simulink model "KalmanFilter"  (R2024a)
settings: Solver=VariableStepAuto  StartTime=0.0  StopTime=10.0  RelTol=1e-3
undefined symbols (not defined in the file or in its folder): Ad, Bd, C, D, GQG, P0, R, x0
libraries: sdl_lib x10, nesl_utility x6, fl_lib x4
settings Model: Creator=Z634594  LastModifiedBy=marisao
settings SolverCC: AlgebraicLoopSolver=TrustRegion
settings DebuggingCC: UnconnectedInputMsg=warning  UnconnectedOutputMsg=warning  UnconnectedLineMsg=warning
settings ModelReferenceCC: EnableRefExpFcnMdlSchedulingChecks=on
settings SFSimCC: CustomCodeUndefinedFunction=UseInterfaceOnly
settings RTWCC: GPUComputeCapability=3.5

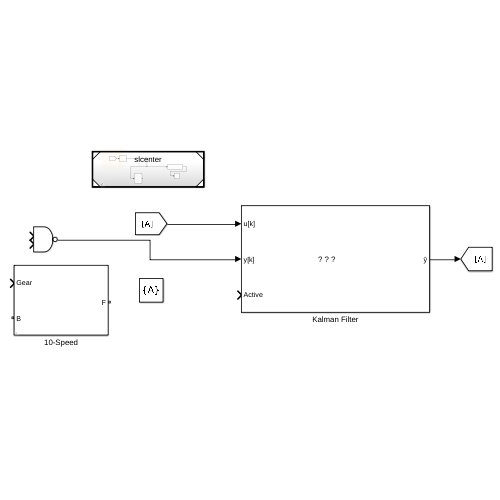
[thumbnail: Simulink's stored preview of the top-level diagram]
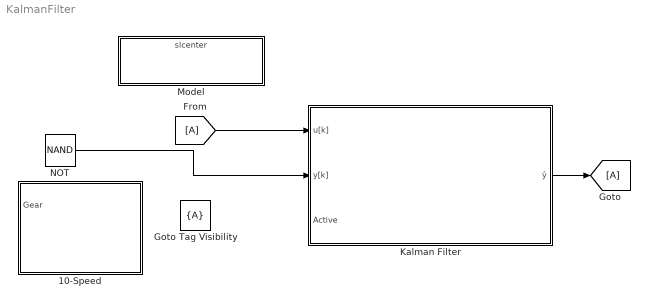
== system KalmanFilter ==
  10-Speed : Subsystem  mask(10-Speed){InitGear=Neutral, ShowInLibBrowser=0, ClutchSchedule={[0 1 1 1 0 1];[0 1 1 0 1 1];[0 1 0 1 1 1];[0 0 1 1 1 1];[1 0 0 1 1 1];[1 0 1 0 1 1];[1 0 1 1 0 1];[1 0 1 1 1 0];[1 1 1 1 0 0];[1 1 0 1 1 0];[1 1 0 1 0 1];[1 1 0 1 0 0]}}
      mask prompts: InitGear "Initial gear"
      mask help: physmod:sdl:library:transmissions:TenSpeed
      mask init:
      | set_param([gcb,'/Clutch A'],'initial_state_locked',num2str(ClutchSchedule{InitGear}(1)));
      | set_param([gcb,'/Clutch B'],'initial_state_locked',num2str(ClutchSchedule{InitGear}(2)));
      | set_param([gcb,'/Clutch C'],'initial_state_locked',num2str(ClutchSchedule{InitGear}(3)));
      | set_param([gcb,'/Clutch D'],'initial_state_locked',num2str(ClutchSchedule{InitGear}(4)));
      | set_param([gcb,'/Clutch E'],'initial_state_locked',num2str(ClutchSchedule{InitGear}(5)));
      | set_param([gcb,'/Clutch F'],'initial_state_locked',num2str(ClutchSchedule{InitGear}(6)));
      mask Help: web([docroot '/sdl/ref/10speed.html'])
      mask TypeOptions InitGear: 10 | 9 | 8 | 7 | 6 | 5 | 4 | 3 | 2 | 1 | physmod:sdl:library:transmissions:Reverse | physmod:sdl:library:transmissions:Neutral
  From : From
  Goto : Goto
  Goto Tag Visibility : GotoTagVisibility
  Kalman Filter : Subsystem
      mask Display: image('C:\Users\Z634594\OneDrive - ZF Friedrichshafen AG\Workspace_MATLAB\14_Tj-Measurement\KalmanFilter\KalmanFilter\img\Kalman.png');
  Model : ModelReference  ModelNameDialog=slcenter.slx  SimulationMode=Normal  ModelReferenceVersion=1.1
  NOT : Logic  Operator=NAND  IconShape=distinctive  AllPortsSameDT=off  OutDataTypeStr=boolean
  wires:
  Kalman Filter/1(ŷ) -> Goto/1
  From/1 -> Kalman Filter/1(u[k])
  NOT/1 -> Kalman Filter/2(y[k])

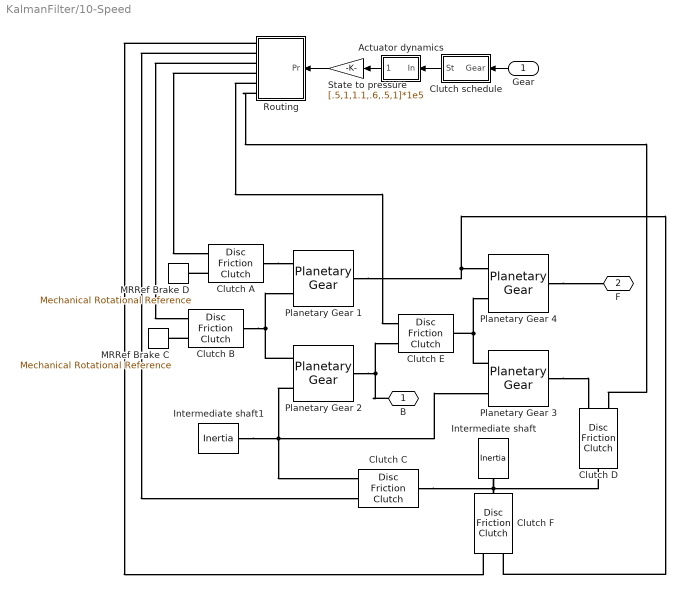
== system KalmanFilter/10-Speed ==
  Gear : Inport
  Actuator dynamics : Subsystem  mask(First-order lag supporting vector signals){b=[1 1 1 1 1 1]*0.05, x_initial=ClutchSchedule{InitGear}}
      mask prompts: b "Filter time constant"; x_initial "Initial output"
      mask help: Models a lag of the form 1/(b*s+1) where s is the Laplace operator.
  Clutch schedule : Subsystem
  Clutch A : sdl_lib/Clutches/Disc Friction Clutch  geometry_model=1  r_eff=130 mm  d_o=150 mm  d_i=100 mm  nS=3  piston_area=0.001 m^2  unidirectional=0  enable_faults=simscape.enum.onoff.off  fault_type=sdl.enum.clutchFault.lock  friction_model=1  mu_w_vector=[0, 100, 1000] rad/s  temperature_TLU=[280, 300, 320] K  mu_static=0.35  mu_static_vector=[.4, .38, .36]  mu_coulomb=0.3  mu_coulomb_vector=[.3, .22, .19]  mu_coulomb_temp_vector=[.3, .28, .25]  mu_coulomb_matrix=[.34, .32, .3; .3, .28, .25; .25, .2, .15]  mu_interp_method=simscape.enum.interpolation.linear  mu_extrap_method=simscape.enum.extrapolation.linear  d_f=1  w_tol=0.001 rad/s  pressure_min=100 Pa  mu_visc=0 N*m/(rad/s)  initial_state_locked=1  thermal_mass=25 kJ/K  T_init=300 K
      settings: InternalSimscapePortConfiguration="{\"Bottom\":[],\"Left\":[{\"id\":\"P\",\"label\":\"P\",\"type\":\"input\"},{\"id\":\"B\",\"label\":\"B\",\"type\":\"foundation.mechanical.rotational.rotational\"}],\"Right\":[{\"id\":\"F\",\"label\":\"F\",\"type\":\"foundation.mechanical.rotational.rotational\"}],\"Top\":[]}"
  Clutch B : sdl_lib/Clutches/Disc Friction Clutch  geometry_model=1  r_eff=130 mm  d_o=150 mm  d_i=100 mm  nS=5  piston_area=0.001 m^2  unidirectional=0  enable_faults=simscape.enum.onoff.off  fault_type=sdl.enum.clutchFault.lock  friction_model=1  mu_w_vector=[0, 100, 1000] rad/s  temperature_TLU=[280, 300, 320] K  mu_static=0.35  mu_static_vector=[.4, .38, .36]  mu_coulomb=0.3  mu_coulomb_vector=[.3, .22, .19]  mu_coulomb_temp_vector=[.3, .28, .25]  mu_coulomb_matrix=[.34, .32, .3; .3, .28, .25; .25, .2, .15]  mu_interp_method=simscape.enum.interpolation.linear  mu_extrap_method=simscape.enum.extrapolation.linear  d_f=1  w_tol=0.001 rad/s  pressure_min=100 Pa  mu_visc=0 N*m/(rad/s)  initial_state_locked=1  thermal_mass=25 kJ/K  T_init=300 K
      settings: InternalSimscapePortConfiguration="{\"Bottom\":[],\"Left\":[{\"id\":\"P\",\"label\":\"P\",\"type\":\"input\"},{\"id\":\"B\",\"label\":\"B\",\"type\":\"foundation.mechanical.rotational.rotational\"}],\"Right\":[{\"id\":\"F\",\"label\":\"F\",\"type\":\"foundation.mechanical.rotational.rotational\"}],\"Top\":[]}"
  Clutch C : sdl_lib/Clutches/Disc Friction Clutch  geometry_model=1  r_eff=130 mm  d_o=150 mm  d_i=100 mm  nS=5  piston_area=0.001 m^2  unidirectional=0  enable_faults=simscape.enum.onoff.off  fault_type=sdl.enum.clutchFault.lock  friction_model=1  mu_w_vector=[0, 100, 1000] rad/s  temperature_TLU=[280, 300, 320] K  mu_static=0.35  mu_static_vector=[.4, .38, .36]  mu_coulomb=0.3  mu_coulomb_vector=[.3, .22, .19]  mu_coulomb_temp_vector=[.3, .28, .25]  mu_coulomb_matrix=[.34, .32, .3; .3, .28, .25; .25, .2, .15]  mu_interp_method=simscape.enum.interpolation.linear  mu_extrap_method=simscape.enum.extrapolation.linear  d_f=1  w_tol=0.001 rad/s  pressure_min=100 Pa  mu_visc=0 N*m/(rad/s)  initial_state_locked=0  thermal_mass=25 kJ/K  T_init=300 K
      settings: InternalSimscapePortConfiguration="{\"Bottom\":[],\"Left\":[{\"id\":\"P\",\"label\":\"P\",\"type\":\"input\"},{\"id\":\"B\",\"label\":\"B\",\"type\":\"foundation.mechanical.rotational.rotational\"}],\"Right\":[{\"id\":\"F\",\"label\":\"F\",\"type\":\"foundation.mechanical.rotational.rotational\"}],\"Top\":[]}"
  Clutch D : sdl_lib/Clutches/Disc Friction Clutch  geometry_model=1  r_eff=130 mm  d_o=150 mm  d_i=100 mm  nS=6  piston_area=0.001 m^2  unidirectional=0  enable_faults=simscape.enum.onoff.off  fault_type=sdl.enum.clutchFault.lock  friction_model=1  mu_w_vector=[0, 100, 1000] rad/s  temperature_TLU=[280, 300, 320] K  mu_static=0.35  mu_static_vector=[.4, .38, .36]  mu_coulomb=0.3  mu_coulomb_vector=[.3, .22, .19]  mu_coulomb_temp_vector=[.3, .28, .25]  mu_coulomb_matrix=[.34, .32, .3; .3, .28, .25; .25, .2, .15]  mu_interp_method=simscape.enum.interpolation.linear  mu_extrap_method=simscape.enum.extrapolation.linear  d_f=1  w_tol=0.001 rad/s  pressure_min=100 Pa  mu_visc=0 N*m/(rad/s)  initial_state_locked=1  thermal_mass=25 kJ/K  T_init=300 K
      settings: InternalSimscapePortConfiguration="{\"Bottom\":[],\"Left\":[{\"id\":\"P\",\"label\":\"P\",\"type\":\"input\"},{\"id\":\"B\",\"label\":\"B\",\"type\":\"foundation.mechanical.rotational.rotational\"}],\"Right\":[{\"id\":\"F\",\"label\":\"F\",\"type\":\"foundation.mechanical.rotational.rotational\"}],\"Top\":[]}"
  Clutch E : sdl_lib/Clutches/Disc Friction Clutch  geometry_model=1  r_eff=130 mm  d_o=150 mm  d_i=100 mm  nS=5  piston_area=0.001 m^2  unidirectional=0  enable_faults=simscape.enum.onoff.off  fault_type=sdl.enum.clutchFault.lock  friction_model=1  mu_w_vector=[0, 100, 1000] rad/s  temperature_TLU=[280, 300, 320] K  mu_static=0.35  mu_static_vector=[.4, .38, .36]  mu_coulomb=0.3  mu_coulomb_vector=[.3, .22, .19]  mu_coulomb_temp_vector=[.3, .28, .25]  mu_coulomb_matrix=[.34, .32, .3; .3, .28, .25; .25, .2, .15]  mu_interp_method=simscape.enum.interpolation.linear  mu_extrap_method=simscape.enum.extrapolation.linear  d_f=1  w_tol=0.001 rad/s  pressure_min=100 Pa  mu_visc=0 N*m/(rad/s)  initial_state_locked=0  thermal_mass=25 kJ/K  T_init=300 K
      settings: InternalSimscapePortConfiguration="{\"Bottom\":[],\"Left\":[{\"id\":\"P\",\"label\":\"P\",\"type\":\"input\"},{\"id\":\"B\",\"label\":\"B\",\"type\":\"foundation.mechanical.rotational.rotational\"}],\"Right\":[{\"id\":\"F\",\"label\":\"F\",\"type\":\"foundation.mechanical.rotational.rotational\"}],\"Top\":[]}"
  Clutch F : sdl_lib/Clutches/Disc Friction Clutch  geometry_model=1  r_eff=130 mm  d_o=150 mm  d_i=100 mm  nS=4  piston_area=0.001 m^2  unidirectional=0  enable_faults=simscape.enum.onoff.off  fault_type=sdl.enum.clutchFault.lock  friction_model=1  mu_w_vector=[0, 100, 1000] rad/s  temperature_TLU=[280, 300, 320] K  mu_static=0.35  mu_static_vector=[.4, .38, .36]  mu_coulomb=0.3  mu_coulomb_vector=[.3, .22, .19]  mu_coulomb_temp_vector=[.3, .28, .25]  mu_coulomb_matrix=[.34, .32, .3; .3, .28, .25; .25, .2, .15]  mu_interp_method=simscape.enum.interpolation.linear  mu_extrap_method=simscape.enum.extrapolation.linear  d_f=1  w_tol=0.001 rad/s  pressure_min=100 Pa  mu_visc=0 N*m/(rad/s)  initial_state_locked=0  thermal_mass=25 kJ/K  T_init=300 K
      settings: InternalSimscapePortConfiguration="{\"Bottom\":[],\"Left\":[{\"id\":\"P\",\"label\":\"P\",\"type\":\"input\"},{\"id\":\"B\",\"label\":\"B\",\"type\":\"foundation.mechanical.rotational.rotational\"}],\"Right\":[{\"id\":\"F\",\"label\":\"F\",\"type\":\"foundation.mechanical.rotational.rotational\"}],\"Top\":[]}"
  Intermediate shaft : fl_lib/Mechanical/Rotational Elements/Inertia  inertia=0.01 kg*m^2  num_ports=foundation.enum.numPorts2.one  w_specify=off  w_priority=High  w=0 rad/s  w_nominal_specify=off  w_nominal_value=1  w_nominal_unit=rad/s  t_specify=off  t_priority=High  t=0 N*m  t_nominal_specify=off  t_nominal_value=1  t_nominal_unit=N*m
  Intermediate shaft1 : fl_lib/Mechanical/Rotational Elements/Inertia  inertia=0.01 kg*m^2  num_ports=foundation.enum.numPorts2.one  w_specify=off  w_priority=High  w=0 rad/s  w_nominal_specify=off  w_nominal_value=1  w_nominal_unit=rad/s  t_specify=off  t_priority=High  t=0 N*m  t_nominal_specify=off  t_nominal_value=1  t_nominal_unit=N*m
  MRRef Brake C : fl_lib/Mechanical/Rotational Elements/Mechanical Rotational Reference
  MRRef Brake D : fl_lib/Mechanical/Rotational Elements/Mechanical Rotational Reference
  Planetary Gear 1 : sdl_lib/Gears/Planetary Gear  rs_ratio=92/44  friction_model=1  efficiency=[ 0.96 0.98 ]  temperature_TLU=[ 280 300 320 ] K  efficiency_sp_TLU=[ 0.95 0.9 0.85 ]  efficiency_rp_TLU=[ 0.95 0.9 0.85 ]  pwr_thr=[ 0.001 0.001 ] W  mu_visc=[ 0 0 ] N*m/(rad/s)  model_inertia=0  planet_inertia=0.001 kg*m^2  thermal_mass=50 J/K  T_init=300 K
  Planetary Gear 2 : sdl_lib/Gears/Planetary Gear  rs_ratio=89/51  friction_model=1  efficiency=[ 0.96 0.98 ]  temperature_TLU=[ 280 300 320 ] K  efficiency_sp_TLU=[ 0.95 0.9 0.85 ]  efficiency_rp_TLU=[ 0.95 0.9 0.85 ]  pwr_thr=[ 0.001 0.001 ] W  mu_visc=[ 0 0 ] N*m/(rad/s)  model_inertia=0  planet_inertia=0.001 kg*m^2  thermal_mass=50 J/K  T_init=300 K
  Planetary Gear 3 : sdl_lib/Gears/Planetary Gear  rs_ratio=101/63  friction_model=1  efficiency=[ 0.96 0.98 ]  temperature_TLU=[ 280 300 320 ] K  efficiency_sp_TLU=[ 0.95 0.9 0.85 ]  efficiency_rp_TLU=[ 0.95 0.9 0.85 ]  pwr_thr=[ 0.001 0.001 ] W  mu_visc=[ 0 0 ] N*m/(rad/s)  model_inertia=0  planet_inertia=0.001 kg*m^2  thermal_mass=50 J/K  T_init=300 K
  Planetary Gear 4 : sdl_lib/Gears/Planetary Gear  rs_ratio=85/23  friction_model=1  efficiency=[ 0.96 0.98 ]  temperature_TLU=[ 280 300 320 ] K  efficiency_sp_TLU=[ 0.95 0.9 0.85 ]  efficiency_rp_TLU=[ 0.95 0.9 0.85 ]  pwr_thr=[ 0.001 0.001 ] W  mu_visc=[ 0 0 ] N*m/(rad/s)  model_inertia=0  planet_inertia=0.001 kg*m^2  thermal_mass=50 J/K  T_init=300 K
  Routing : Subsystem
  State to pressure : Gain  Gain=[.5,1,1.1,.6,.5,1]*1e5
  B : PMIOPort  Side=Left
  F : PMIOPort  Port=2  Side=Right
  wires:
  Gear/1 -> Clutch schedule/1(Gear)
  Clutch schedule/1(St) -> Actuator dynamics/1(In)
  State to pressure/1 -> Routing/1(Pr)
  Actuator dynamics/1(Out) -> State to pressure/1
  connections:
  Clutch A/LConn2 -- MRRef Brake D/LConn1
  Clutch B/LConn2 -- MRRef Brake C/LConn1
  Planetary Gear 4/LConn1 -- F/RConn1
  B/RConn1 -- Planetary Gear 2/LConn1 -- Clutch E/LConn2
  Clutch A/RConn1 -- Planetary Gear 1/RConn1
  Clutch B/RConn1 -- Planetary Gear 2/RConn2 -- Planetary Gear 1/RConn2
  Planetary Gear 1/LConn1 -- Planetary Gear 4/RConn1 -- Clutch F/LConn2
  Planetary Gear 2/RConn1 -- Intermediate shaft1/LConn1 -- Planetary Gear 3/RConn2 -- Clutch C/LConn2
  Planetary Gear 3/RConn1 -- Planetary Gear 4/RConn2 -- Clutch E/RConn1
  Planetary Gear 3/LConn1 -- Clutch D/LConn2
  Clutch F/RConn1 -- Clutch C/RConn1 -- Intermediate shaft/LConn1 -- Clutch D/RConn1
  Routing/RConn1 -- Clutch F/LConn1
  Routing/RConn2 -- Clutch C/LConn1
  Routing/RConn3 -- Clutch B/LConn1
  Routing/RConn4 -- Clutch A/LConn1
  Routing/RConn5 -- Clutch E/LConn1
  Routing/RConn6 -- Clutch D/LConn1

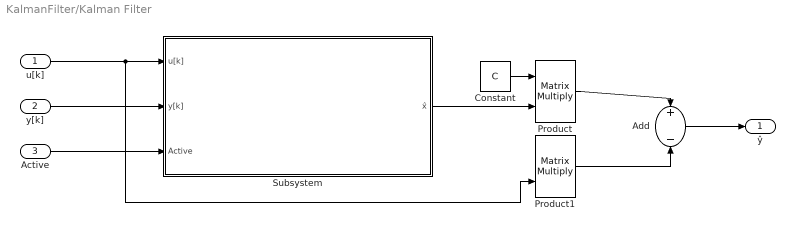
== system KalmanFilter/Kalman Filter ==
  u[k] : Inport
  y[k] : Inport  Port=2
  Active : Inport  Port=3
  Add : Sum  Inputs=+-
  Constant : Constant  Value=C  VectorParams1D=off
  Product : Product  Multiplication=Matrix(*)
  Product1 : Product  Multiplication=Matrix(*)
  Subsystem : Subsystem
      mask Display: image('C:\Users\Z634594\OneDrive - ZF Friedrichshafen AG\Workspace_MATLAB\14_Tj-Measurement\KalmanFilter\KalmanFilter\img\KalmanEquations.jpg');
  ŷ : Outport  VectorParamsAs1DForOutWhenUnconnected=off
  wires:
  u[k]/1 -> Product1/2, Subsystem/1(u[k])
  y[k]/1 -> Subsystem/2(y[k])
  ? -> Product1/1
  Product/1 -> Add/1
  Constant/1 -> Product/1
  Subsystem/1(x̂) -> Product/2
  Add/1 -> ŷ/1
  Product1/1 -> Add/2
  Active/1 -> Subsystem/3(Active)

== system KalmanFilter/10-Speed/Actuator dynamics ==
  In : Inport
  Gain : Gain  Gain=1./b
  Integrator : Integrator  InitialCondition=x_initial.*b
  Sum : Sum  Inputs=|+-  InputSameDT=on  SaturateOnIntegerOverflow=on  OutDataTypeStr=Inherit: Same as first input
  Out : Outport  VectorParamsAs1DForOutWhenUnconnected=off
  wires:
  Gain/1 -> Out/1, Sum/2
  Integrator/1 -> Gain/1
  In/1 -> Sum/1
  Sum/1 -> Integrator/1

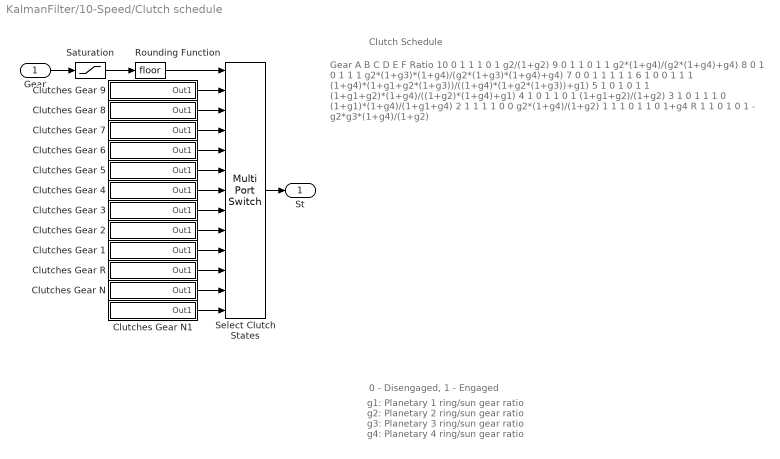
== system KalmanFilter/10-Speed/Clutch schedule ==
  note: Clutch Schedule
  note: Gear
      | A
      | B
      | C
      | D
      | E
      | F
      | Ratio
      |
      | 10
      | 0
      | 1
      | 1
      | 1
      | 0
      | 1
      | g2/(1+g2)
      |
      | 9
      | 0
      | 1
      | 1
      | 0
      | 1
      | 1
      | g2*(1+g4)/(g2*(1+g4)+g4)
      |
      | 8
      | 0
      | 1
      | 0
      | 1
      | 1
      | 1
      | g2*(1+g3)*(1+g4)/(g2*(1+g3)*(1+g4)+g4)
      |
      | 7
      | 0
      | 0
      | 1
      | 1
      | 1
      | 1
      | 1
      |
      | 6
      | 1
      | 0
      | 0
      | 1
      | 1
      | 1
      | (1+g4)*(1+g1+g2*(1+g3))/((1+g4)*(1+g2*(1+g3))+g1)
      |
      | 5
      | 1
      | 0
      | 1
      | 0
      | 1
      | 1
      | (1+g1+g2)*(1+g4)/((1+g2)*(1+g4)+g1)
      |
      | 4
      | 1
      | 0
      | 1
      | 1
      | 0
      | 1
      | (1+g1+g2)/(1+g2)
      |
      | 3
      | 1
      | 0
      | 1
      | 1
      | 1
      | 0
      | (1+g1)*(1+g4)/(1+g1+g4)
      |
      | 2
      | 1
      | 1
      | 1
      | 1
      | 0
      | 0
      | g2*(1+g4)/(1+g2)
      |
      | 1
      | 1
      | 1
      | 0
      | 1
      | 1
      | 0
      | 1+g4
      |
      | R
      | 1
      | 1
      | 0
      | 1
      | 0
      | 1
      | - g2*g3*(1+g4)/(1+g2)
  note: 0 - Disengaged, 1 - Engaged
  note: g1: Planetary 1 ring/sun gear ratio
      | g2: Planetary 2 ring/sun gear ratio
      | g3: Planetary 3 ring/sun gear ratio
      | g4: Planetary 4 ring/sun gear ratio
  Gear : Inport
  Clutches Gear 1 : Subsystem  mask{Clutches=ClutchSchedule{9}}
      settings: OpenFcn=open_system(gcb,'force');
      mask Display: disp(Clutches)
  Clutches Gear 2 : Subsystem  mask{Clutches=ClutchSchedule{8}}
      settings: OpenFcn=open_system(gcb,'force');
      mask Display: disp(Clutches)
  Clutches Gear 3 : Subsystem  mask{Clutches=ClutchSchedule{7}}
      settings: OpenFcn=open_system(gcb,'force');
      mask Display: disp(Clutches)
  Clutches Gear 4 : Subsystem  mask{Clutches=ClutchSchedule{6}}
      settings: OpenFcn=open_system(gcb,'force');
      mask Display: disp(Clutches)
  Clutches Gear 5 : Subsystem  mask{Clutches=ClutchSchedule{5}}
      settings: OpenFcn=open_system(gcb,'force');
      mask Display: disp(Clutches)
  Clutches Gear 6 : Subsystem  mask{Clutches=ClutchSchedule{4}}
      settings: OpenFcn=open_system(gcb,'force');
      mask Display: disp(Clutches)
  Clutches Gear 7 : Subsystem  mask{Clutches=ClutchSchedule{3}}
      settings: OpenFcn=open_system(gcb,'force');
      mask Display: disp(Clutches)
  Clutches Gear 8 : Subsystem  mask{Clutches=ClutchSchedule{2}}
      settings: OpenFcn=open_system(gcb,'force');
      mask Display: disp(Clutches)
  Clutches Gear 9 : Subsystem  mask{Clutches=ClutchSchedule{1}}
      settings: OpenFcn=open_system(gcb,'force');
      mask Display: disp(Clutches)
  Clutches Gear N : Subsystem  mask{Clutches=ClutchSchedule{11}}
      settings: OpenFcn=open_system(gcb,'force');
      mask Display: disp(Clutches)
  Clutches Gear N1 : Subsystem  mask{Clutches=ClutchSchedule{12}}
      settings: OpenFcn=open_system(gcb,'force');
      mask Display: disp(Clutches)
  Clutches Gear R : Subsystem  mask{Clutches=ClutchSchedule{10}}
      settings: OpenFcn=open_system(gcb,'force');
      mask Display: disp(Clutches)
  Rounding Function : Rounding
  Saturation : Saturate  UpperLimit=10  LowerLimit=-1  ZeroCross=off
  Select Clutch States : MultiPortSwitch  DataPortOrder=Specify indices  DataPortIndices={10,9,8,7,6,5,4,3,2,1,-1,0}  DiagnosticForDefault=None  SaturateOnIntegerOverflow=off  InputSameDT=off
  St : Outport  VectorParamsAs1DForOutWhenUnconnected=off
  wires:
  Select Clutch States/1 -> St/1
  Rounding Function/1 -> Select Clutch States/1
  Saturation/1 -> Rounding Function/1
  Clutches Gear N/1(Out1) -> Select Clutch States/12
  Clutches Gear R/1(Out1) -> Select Clutch States/11
  Clutches Gear 3/1(Out1) -> Select Clutch States/8
  Clutches Gear 2/1(Out1) -> Select Clutch States/9
  Clutches Gear 1/1(Out1) -> Select Clutch States/10
  Clutches Gear 8/1(Out1) -> Select Clutch States/3
  Clutches Gear 5/1(Out1) -> Select Clutch States/6
  Clutches Gear 4/1(Out1) -> Select Clutch States/7
  Clutches Gear 6/1(Out1) -> Select Clutch States/5
  Clutches Gear 7/1(Out1) -> Select Clutch States/4
  Clutches Gear 9/1(Out1) -> Select Clutch States/2
  Gear/1 -> Saturation/1
  Clutches Gear N1/1(Out1) -> Select Clutch States/13

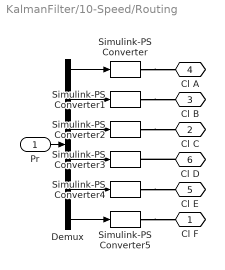
== system KalmanFilter/10-Speed/Routing ==
  Pr : Inport
  Demux : Demux  Outputs=6
  Simulink-PS Converter{,1..5} (6 alike) : nesl_utility/Simulink-PS Converter  PhysicalDomain=network_engine_domain  SubClassName=ps_input  LeftPortType=input  RightPortType=output  PseudoPeriodic=off  Frequencies=[]  NoiseDistribution=none  NoiseParameters=[]  Unit=1  AffineConversion=off  FilteringAndDerivatives=zero  SimscapeFilterOrder=1  InputFilterTimeConstant=0.001  UdotUserProvided=1
  Cl F : PMIOPort  Side=Right
  Cl C : PMIOPort  Port=2  Side=Right
  Cl B : PMIOPort  Port=3  Side=Right
  Cl A : PMIOPort  Port=4  Side=Right
  Cl E : PMIOPort  Port=5  Side=Right
  Cl D : PMIOPort  Port=6  Side=Right
  wires:
  Demux/6 -> Simulink-PS Converter5/1
  Demux/5 -> Simulink-PS Converter4/1
  Demux/4 -> Simulink-PS Converter3/1
  Demux/3 -> Simulink-PS Converter2/1
  Demux/2 -> Simulink-PS Converter1/1
  Demux/1 -> Simulink-PS Converter/1
  Pr/1 -> Demux/1
  connections:
  Simulink-PS Converter2/RConn1 -- Cl C/RConn1
  Simulink-PS Converter/RConn1 -- Cl A/RConn1
  Simulink-PS Converter1/RConn1 -- Cl B/RConn1
  Cl D/RConn1 -- Simulink-PS Converter3/RConn1
  Simulink-PS Converter4/RConn1 -- Cl E/RConn1
  Simulink-PS Converter5/RConn1 -- Cl F/RConn1

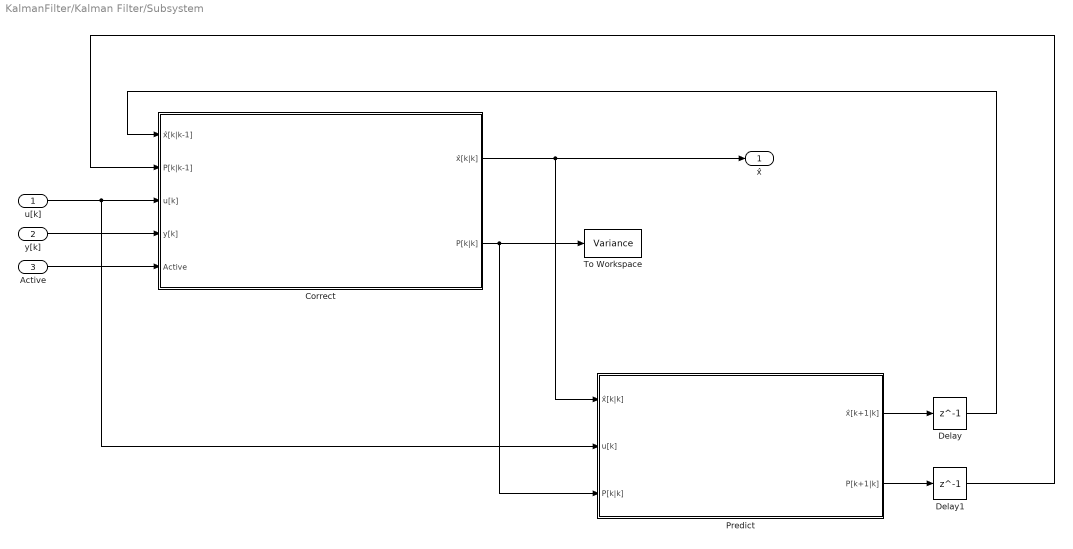
== system KalmanFilter/Kalman Filter/Subsystem ==
  u[k] : Inport
  y[k] : Inport  Port=2
  Active : Inport  Port=3
  Correct : Subsystem
      mask Display: image('C:\Users\Z634594\OneDrive - ZF Friedrichshafen AG\Workspace_MATLAB\14_Tj-Measurement\KalmanFilter\KalmanFilter\img\Update.png');
  Delay : Delay  DelayLength=1  InitialCondition=x0
  Delay1 : Delay  DelayLength=1  InitialCondition=P0
  Predict : Subsystem
      mask Display: image('C:\Users\Z634594\OneDrive - ZF Friedrichshafen AG\Workspace_MATLAB\14_Tj-Measurement\Simulink\img\Predict.png');
  To Workspace : ToWorkspace  VariableName=Variance  SampleTime=-1
      settings: MaxDataPoints=1
  x̂ : Outport  VectorParamsAs1DForOutWhenUnconnected=off
  wires:
  Predict/1(x̂[k+1|k]) -> Delay/1
  Delay/1 -> Correct/1(x̂[k|k-1])
  Predict/2(P[k+1|k]) -> Delay1/1
  Delay1/1 -> Correct/2(P[k|k-1])
  Correct/1(x̂[k|k]) -> x̂/1, Predict/1(x̂[k|k])
  Correct/2(P[k|k]) -> To Workspace/1, Predict/3(P[k|k])
  u[k]/1 -> Correct/3(u[k]), Predict/2(u[k])
  y[k]/1 -> Correct/4(y[k])
  Active/1 -> Correct/5(Active)

== system KalmanFilter/10-Speed/Clutch schedule/Clutches Gear 1 ==
  Clutches : Constant  Value=Clutches  SampleTime=0
  Out1 : Outport  VectorParamsAs1DForOutWhenUnconnected=off
  wires:
  Clutches/1 -> Out1/1

== system KalmanFilter/10-Speed/Clutch schedule/Clutches Gear 2 ==
  Clutches : Constant  Value=Clutches  SampleTime=0
  Out1 : Outport  VectorParamsAs1DForOutWhenUnconnected=off
  wires:
  Clutches/1 -> Out1/1

== system KalmanFilter/10-Speed/Clutch schedule/Clutches Gear 3 ==
  Clutches : Constant  Value=Clutches  SampleTime=0
  Out1 : Outport  VectorParamsAs1DForOutWhenUnconnected=off
  wires:
  Clutches/1 -> Out1/1

== system KalmanFilter/10-Speed/Clutch schedule/Clutches Gear 4 ==
  Clutches : Constant  Value=Clutches  SampleTime=0
  Out1 : Outport  VectorParamsAs1DForOutWhenUnconnected=off
  wires:
  Clutches/1 -> Out1/1

== system KalmanFilter/10-Speed/Clutch schedule/Clutches Gear 5 ==
  Clutches : Constant  Value=Clutches  SampleTime=0
  Out1 : Outport  VectorParamsAs1DForOutWhenUnconnected=off
  wires:
  Clutches/1 -> Out1/1

== system KalmanFilter/10-Speed/Clutch schedule/Clutches Gear 6 ==
  Clutches : Constant  Value=Clutches  SampleTime=0
  Out1 : Outport  VectorParamsAs1DForOutWhenUnconnected=off
  wires:
  Clutches/1 -> Out1/1

== system KalmanFilter/10-Speed/Clutch schedule/Clutches Gear 7 ==
  Clutches : Constant  Value=Clutches  SampleTime=0
  Out1 : Outport  VectorParamsAs1DForOutWhenUnconnected=off
  wires:
  Clutches/1 -> Out1/1

== system KalmanFilter/10-Speed/Clutch schedule/Clutches Gear 8 ==
  Clutches : Constant  Value=Clutches  SampleTime=0
  Out1 : Outport  VectorParamsAs1DForOutWhenUnconnected=off
  wires:
  Clutches/1 -> Out1/1

== system KalmanFilter/10-Speed/Clutch schedule/Clutches Gear 9 ==
  Clutches : Constant  Value=Clutches  SampleTime=0
  Out1 : Outport  VectorParamsAs1DForOutWhenUnconnected=off
  wires:
  Clutches/1 -> Out1/1

== system KalmanFilter/10-Speed/Clutch schedule/Clutches Gear N ==
  Clutches Gear N : Constant  Value=Clutches  SampleTime=0
  Out1 : Outport  VectorParamsAs1DForOutWhenUnconnected=off
  wires:
  Clutches Gear N/1 -> Out1/1

== system KalmanFilter/10-Speed/Clutch schedule/Clutches Gear N1 ==
  Clutches Gear N : Constant  Value=Clutches  SampleTime=0
  Out1 : Outport  VectorParamsAs1DForOutWhenUnconnected=off
  wires:
  Clutches Gear N/1 -> Out1/1

== system KalmanFilter/10-Speed/Clutch schedule/Clutches Gear R ==
  Clutches : Constant  Value=Clutches  SampleTime=0
  Out1 : Outport  VectorParamsAs1DForOutWhenUnconnected=off
  wires:
  Clutches/1 -> Out1/1

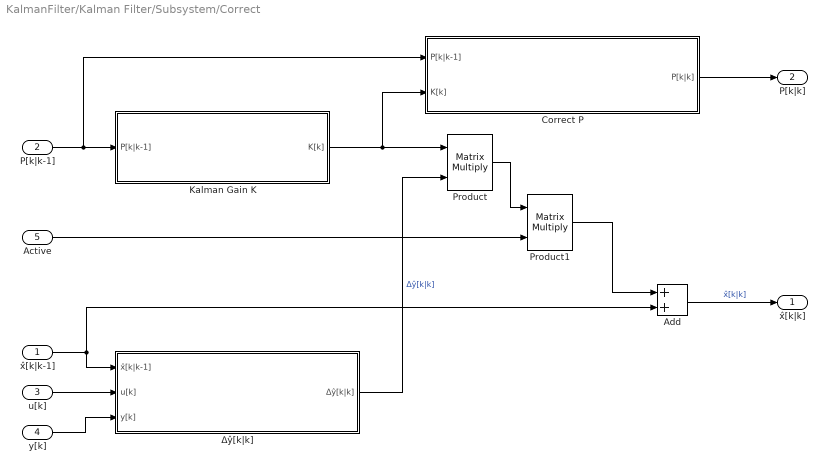
== system KalmanFilter/Kalman Filter/Subsystem/Correct ==
  x̂[k|k-1] : Inport
  P[k|k-1] : Inport  Port=2
  u[k] : Inport  Port=3
  y[k] : Inport  Port=4
  Active : Inport  Port=5
  Add : Sum
  Correct P : Subsystem
      mask Display: image('C:\Users\Z634594\OneDrive - ZF Friedrichshafen AG\Workspace_MATLAB\14_Tj-Measurement\KalmanFilter\KalmanFilter\img\UpdateP.png');
  Kalman Gain K : Subsystem
      mask Display: image('C:\Users\Z634594\OneDrive - ZF Friedrichshafen AG\Workspace_MATLAB\14_Tj-Measurement\KalmanFilter\KalmanFilter\img\UpdateK.png');
  Product : Product  Multiplication=Matrix(*)
  Product1 : Product  Multiplication=Matrix(*)
  Δŷ[k|k] : Subsystem
      mask Display: image('C:\Users\Z634594\OneDrive - ZF Friedrichshafen AG\Workspace_MATLAB\14_Tj-Measurement\KalmanFilter\KalmanFilter\img\CalcdeltaY.png');
  x̂[k|k] : Outport  VectorParamsAs1DForOutWhenUnconnected=off
  P[k|k] : Outport  Port=2  VectorParamsAs1DForOutWhenUnconnected=off
  wires:
  x̂[k|k-1]/1 -> Δŷ[k|k]/1(x̂[k|k-1]), Add/2
  Add/1 -> x̂[k|k]/1  "x̂[k|k]"
  Δŷ[k|k]/1(Δŷ[k|k]) -> Product/2  "Δŷ[k|k]"
  Kalman Gain K/1(K[k]) -> Correct P/2(K[k]), Product/1
  P[k|k-1]/1 -> Correct P/1(P[k|k-1]), Kalman Gain K/1(P[k|k-1])
  Correct P/1(P[k|k]) -> P[k|k]/1
  u[k]/1 -> Δŷ[k|k]/2(u[k])
  y[k]/1 -> Δŷ[k|k]/3(y[k])
  Product/1 -> Product1/1
  Product1/1 -> Add/1
  Active/1 -> Product1/2

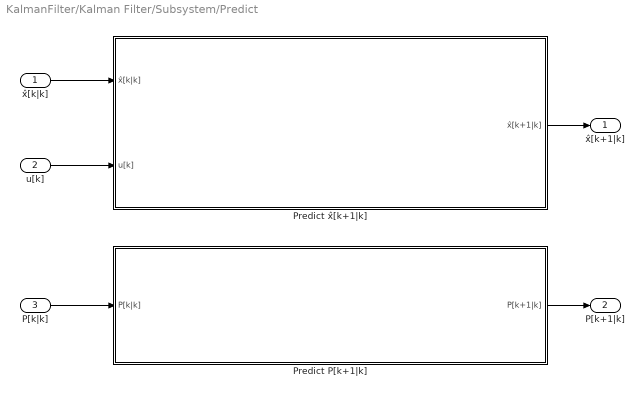
== system KalmanFilter/Kalman Filter/Subsystem/Predict ==
  x̂[k|k] : Inport
  u[k] : Inport  Port=2
  P[k|k] : Inport  Port=3
  Predict P[k+1|k] : Subsystem
      mask Display: image('C:\Users\Z634594\OneDrive - ZF Friedrichshafen AG\Workspace_MATLAB\14_Tj-Measurement\KalmanFilter\KalmanFilter\img\PredictP.png');
  Predict x̂[k+1|k] : Subsystem
      mask Display: image('C:\Users\Z634594\OneDrive - ZF Friedrichshafen AG\Workspace_MATLAB\14_Tj-Measurement\KalmanFilter\KalmanFilter\img\Predictx.png');
  x̂[k+1|k] : Outport  VectorParamsAs1DForOutWhenUnconnected=off
  P[k+1|k] : Outport  Port=2  VectorParamsAs1DForOutWhenUnconnected=off
  wires:
  u[k]/1 -> Predict x̂[k+1|k]/2(u[k])
  x̂[k|k]/1 -> Predict x̂[k+1|k]/1(x̂[k|k])
  Predict x̂[k+1|k]/1(x̂[k+1|k]) -> x̂[k+1|k]/1
  Predict P[k+1|k]/1(P[k+1|k]) -> P[k+1|k]/1
  P[k|k]/1 -> Predict P[k+1|k]/1(P[k|k])

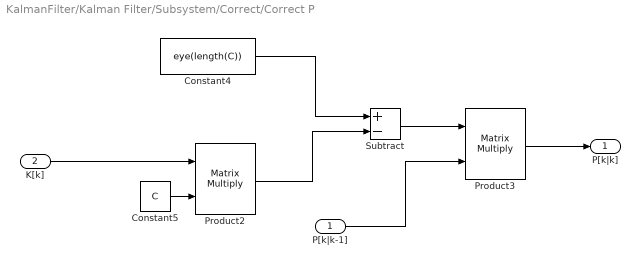
== system KalmanFilter/Kalman Filter/Subsystem/Correct/Correct P ==
  P[k|k-1] : Inport
  K[k] : Inport  Port=2
  Constant4 : Constant  Value=eye(length(C))  VectorParams1D=off
  Constant5 : Constant  Value=C  VectorParams1D=off
  Product2 : Product  Multiplication=Matrix(*)
  Product3 : Product  Multiplication=Matrix(*)
  Subtract : Sum  Inputs=+-
  P[k|k] : Outport  VectorParamsAs1DForOutWhenUnconnected=off
  wires:
  Constant5/1 -> Product2/2
  Constant4/1 -> Subtract/1
  Product2/1 -> Subtract/2
  P[k|k-1]/1 -> Product3/2
  K[k]/1 -> Product2/1
  Subtract/1 -> Product3/1
  Product3/1 -> P[k|k]/1

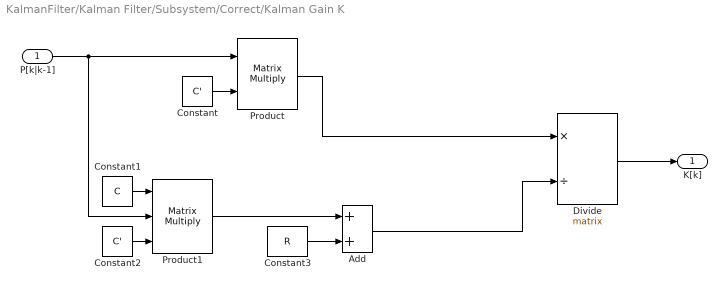
== system KalmanFilter/Kalman Filter/Subsystem/Correct/Kalman Gain K ==
  P[k|k-1] : Inport
  Add : Sum
  Constant : Constant  Value=C'  VectorParams1D=off
  Constant1 : Constant  Value=C  VectorParams1D=off
  Constant2 : Constant  Value=C'  VectorParams1D=off
  Constant3 : Constant  Value=R  VectorParams1D=off
  Divide : Product  Inputs=*/  Multiplication=Matrix(*)
  Product : Product  Multiplication=Matrix(*)
  Product1 : Product  Inputs=3  Multiplication=Matrix(*)
  K[k] : Outport  VectorParamsAs1DForOutWhenUnconnected=off
  wires:
  Constant/1 -> Product/2
  Product/1 -> Divide/1
  Constant1/1 -> Product1/1
  Divide/1 -> K[k]/1
  Constant3/1 -> Add/2
  Add/1 -> Divide/2
  Product1/1 -> Add/1
  P[k|k-1]/1 -> Product1/2, Product/1
  Constant2/1 -> Product1/3

== system KalmanFilter/Kalman Filter/Subsystem/Correct/Δŷ[k|k] ==
  x̂[k|k-1] : Inport
  u[k] : Inport  Port=2
  y[k] : Inport  Port=3
  Calculate ŷ[k|k-1] : Subsystem
      mask Display: image('C:\Users\Z634594\OneDrive - ZF Friedrichshafen AG\Workspace_MATLAB\14_Tj-Measurement\Simulink\img\Calcy.png');
  Scope : Scope
  Subtract : Sum  Inputs=+-
  Δŷ[k|k] : Outport  VectorParamsAs1DForOutWhenUnconnected=off
  wires:
  x̂[k|k-1]/1 -> Calculate ŷ[k|k-1]/1(x̂[k|k-1])
  u[k]/1 -> Calculate ŷ[k|k-1]/2(u[k])
  y[k]/1 -> Subtract/1
  Calculate ŷ[k|k-1]/1(ŷ[k|k-1]) -> Scope/1, Subtract/2
  Subtract/1 -> Δŷ[k|k]/1

== system KalmanFilter/Kalman Filter/Subsystem/Predict/Predict P[k+1|k] ==
  P[k|k] : Inport
  Add : Sum
  Constant : Constant  Value=Ad  VectorParams1D=off
  Constant1 : Constant  Value=GQG  VectorParams1D=off
  Constant2 : Constant  Value=Ad'  VectorParams1D=off
  Product : Product  Inputs=3  Multiplication=Matrix(*)
  P[k+1|k] : Outport  VectorParamsAs1DForOutWhenUnconnected=off
  wires:
  Constant/1 -> Product/1
  P[k|k]/1 -> Product/2
  Constant2/1 -> Product/3
  Product/1 -> Add/1
  Constant1/1 -> Add/2
  Add/1 -> P[k+1|k]/1

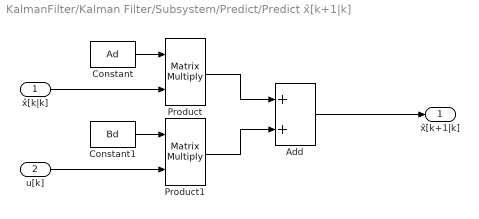
== system KalmanFilter/Kalman Filter/Subsystem/Predict/Predict x̂[k+1|k] ==
  x̂[k|k] : Inport
  u[k] : Inport  Port=2
  Add : Sum
  Constant : Constant  Value=Ad  VectorParams1D=off
  Constant1 : Constant  Value=Bd  VectorParams1D=off
  Product : Product  Multiplication=Matrix(*)
  Product1 : Product  Multiplication=Matrix(*)
  x̂[k+1|k] : Outport  VectorParamsAs1DForOutWhenUnconnected=off
  wires:
  x̂[k|k]/1 -> Product/2
  Add/1 -> x̂[k+1|k]/1
  Constant/1 -> Product/1
  Product/1 -> Add/1
  u[k]/1 -> Product1/2
  Constant1/1 -> Product1/1
  Product1/1 -> Add/2

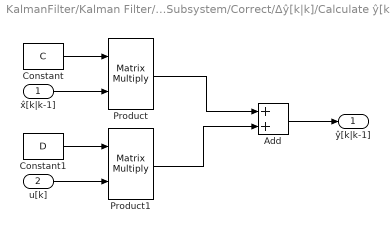
== system KalmanFilter/Kalman Filter/Subsystem/Correct/Δŷ[k|k]/Calculate ŷ[k|k-1] ==
  x̂[k|k-1] : Inport
  u[k] : Inport  Port=2
  Add : Sum
  Constant : Constant  Value=C  VectorParams1D=off
  Constant1 : Constant  Value=D  VectorParams1D=off
  Product : Product  Multiplication=Matrix(*)
  Product1 : Product  Multiplication=Matrix(*)
  ŷ[k|k-1] : Outport  VectorParamsAs1DForOutWhenUnconnected=off
  wires:
  u[k]/1 -> Product1/2
  Product/1 -> Add/1
  x̂[k|k-1]/1 -> Product/2
  Constant/1 -> Product/1
  Constant1/1 -> Product1/1
  Add/1 -> ŷ[k|k-1]/1
  Product1/1 -> Add/2
